simulink model "ieee80211n"  (Simulink 6.0)
settings: Solver=VariableStepDiscrete  StartTime=0.0  StopTime=inf  RelTol=1e-3
PreLoadFcn:
  | load IEEE80211n_init;
values from neighbouring files (symbols this model uses):
  params =     [IEEE80211n_init.mat]    (also in IEEE80211n_settings.m = p)
undefined symbols (not defined in the file or in its folder): magnitude
libraries: commblkintrlv2 x196, dspsigops x143, simulink x136, commdigbbndam2 x98, dspmtrx3 x96, dspsigattribs x69, dspstat3 x38, commutil2 x32, commsequence2 x26, commcnvcod2 x10, dspindex x9, dspmlti3 x8
(part 12 of 12)

== system ieee80211n/MIMODetection/Channel Estimation/ChannelEst6/Channel estimates ==
  trn : Inport  Port=1  LatchInput=off
  in : Inport  Port=2  LatchInput=off
  Enable Averaging : MultiPortSwitch  Inputs=2  zeroidx=on  SaturateOnIntegerOverflow=on
  Enable Averaging1 : MultiPortSwitch  Inputs=2  zeroidx=on  SaturateOnIntegerOverflow=on
  Frame Status Conversion1 : dspsigattribs/Frame Status Conversion  growRefPort=off  outframe=Frame-based
  Mean2 : dspstat3/Mean  DialogController=dspDDGCreate  DialogControllerArgs=DataTag27  run=off  reset_popup=None  roundingMode=Floor  overflowMode=off
  Mean3 : dspstat3/Mean  DialogController=dspDDGCreate  DialogControllerArgs=DataTag28  run=off  reset_popup=None  roundingMode=Floor  overflowMode=off
  Nsts > 1 : Constant  Value=params.NSTS > 1
  One sym only (in) : S-Function  AncestorBlock=dspindex/Multiport Selector  FunctionName=sdspmultiportsel  Parameters=rowsOrCols, numOutports, flatIdxVect, flatLenVect, idxErrMode  mask(Multiport Selector){rowsOrCols=Rows, idxCellArray=1, idxErrMode=Clip Index}
      mask prompts: rowsOrCols "Select:"; idxCellArray "Indices to output:"; idxErrMode "Invalid index:"
      mask help: Output specified rows or columns to one or more output ports. The number of output ports is determined by the number of index vectors, each specified as a separate vector entry in a cell array. Indices are 1-based and need not be unique.
      mask init:
      | [numOutports, flatLenVect, flatIdxVect] = dspblkmultiportsel(idxCellArray);
      mask Help: web(dspbhelp);
      mask StyleString: popup(Rows|Columns),edit,popup(Clip Index|Clip and Warn|Generate Error)
      mask Display: disp(['Select\n' &1]);
  One sym only (trn) : S-Function  AncestorBlock=dspindex/Multiport Selector  FunctionName=sdspmultiportsel  Parameters=rowsOrCols, numOutports, flatIdxVect, flatLenVect, idxErrMode  mask(Multiport Selector){rowsOrCols=Rows, idxCellArray=1, idxErrMode=Clip Index}
      mask prompts: rowsOrCols "Select:"; idxCellArray "Indices to output:"; idxErrMode "Invalid index:"
      mask help: Output specified rows or columns to one or more output ports. The number of output ports is determined by the number of index vectors, each specified as a separate vector entry in a cell array. Indices are 1-based and need not be unique.
      mask init:
      | [numOutports, flatLenVect, flatIdxVect] = dspblkmultiportsel(idxCellArray);
      mask Help: web(dspbhelp);
      mask StyleString: popup(Rows|Columns),edit,popup(Clip Index|Clip and Warn|Generate Error)
      mask Display: disp(['Select\n' &1]);
  Product2 : Product  Inputs=**  SaturateOnIntegerOverflow=on
  Product4 : Product  Inputs=/*  SaturateOnIntegerOverflow=on
  Transpose : dspmtrx3/Transpose  Hermitian=off  overflowFlag=on
  Transpose1 : dspmtrx3/Transpose  Hermitian=off  overflowFlag=on
  Transpose2 : dspmtrx3/Transpose  Hermitian=off  overflowFlag=on
  ch est : Outport
  wires:
  trn/1 -> Transpose/1
  Product4/1 -> Frame Status Conversion1/1
  Frame Status Conversion1/1 -> Transpose1/1
  Transpose1/1 -> ch est/1
  in/1 -> Transpose2/1
  Mean2/1 -> Enable Averaging/3
  Mean3/1 -> Enable Averaging1/3
  Transpose/1 -> Product2/1, Product2/2
  Transpose2/1 -> Mean3/1, One sym only (in)/1
  Product2/1 -> Mean2/1, One sym only (trn)/1
  Enable Averaging/1 -> Product4/1
  Nsts > 1/1 -> Enable Averaging/1, Enable Averaging1/1
  One sym only (in)/1 -> Enable Averaging1/2
  Enable Averaging1/1 -> Product4/2
  One sym only (trn)/1 -> Enable Averaging/2

== system ieee80211n/MIMODetection/Channel Estimation/ChannelEst7/Channel estimates ==
  trn : Inport  Port=1  LatchInput=off
  in : Inport  Port=2  LatchInput=off
  Enable Averaging : MultiPortSwitch  Inputs=2  zeroidx=on  SaturateOnIntegerOverflow=on
  Enable Averaging1 : MultiPortSwitch  Inputs=2  zeroidx=on  SaturateOnIntegerOverflow=on
  Frame Status Conversion1 : dspsigattribs/Frame Status Conversion  growRefPort=off  outframe=Frame-based
  Mean2 : dspstat3/Mean  DialogController=dspDDGCreate  DialogControllerArgs=DataTag29  run=off  reset_popup=None  roundingMode=Floor  overflowMode=off
  Mean3 : dspstat3/Mean  DialogController=dspDDGCreate  DialogControllerArgs=DataTag30  run=off  reset_popup=None  roundingMode=Floor  overflowMode=off
  Nsts > 1 : Constant  Value=params.NSTS > 1
  One sym only (in) : S-Function  AncestorBlock=dspindex/Multiport Selector  FunctionName=sdspmultiportsel  Parameters=rowsOrCols, numOutports, flatIdxVect, flatLenVect, idxErrMode  mask(Multiport Selector){rowsOrCols=Rows, idxCellArray=1, idxErrMode=Clip Index}
      mask prompts: rowsOrCols "Select:"; idxCellArray "Indices to output:"; idxErrMode "Invalid index:"
      mask help: Output specified rows or columns to one or more output ports. The number of output ports is determined by the number of index vectors, each specified as a separate vector entry in a cell array. Indices are 1-based and need not be unique.
      mask init:
      | [numOutports, flatLenVect, flatIdxVect] = dspblkmultiportsel(idxCellArray);
      mask Help: web(dspbhelp);
      mask StyleString: popup(Rows|Columns),edit,popup(Clip Index|Clip and Warn|Generate Error)
      mask Display: disp(['Select\n' &1]);
  One sym only (trn) : S-Function  AncestorBlock=dspindex/Multiport Selector  FunctionName=sdspmultiportsel  Parameters=rowsOrCols, numOutports, flatIdxVect, flatLenVect, idxErrMode  mask(Multiport Selector){rowsOrCols=Rows, idxCellArray=1, idxErrMode=Clip Index}
      mask prompts: rowsOrCols "Select:"; idxCellArray "Indices to output:"; idxErrMode "Invalid index:"
      mask help: Output specified rows or columns to one or more output ports. The number of output ports is determined by the number of index vectors, each specified as a separate vector entry in a cell array. Indices are 1-based and need not be unique.
      mask init:
      | [numOutports, flatLenVect, flatIdxVect] = dspblkmultiportsel(idxCellArray);
      mask Help: web(dspbhelp);
      mask StyleString: popup(Rows|Columns),edit,popup(Clip Index|Clip and Warn|Generate Error)
      mask Display: disp(['Select\n' &1]);
  Product2 : Product  Inputs=**  SaturateOnIntegerOverflow=on
  Product4 : Product  Inputs=/*  SaturateOnIntegerOverflow=on
  Transpose : dspmtrx3/Transpose  Hermitian=off  overflowFlag=on
  Transpose1 : dspmtrx3/Transpose  Hermitian=off  overflowFlag=on
  Transpose2 : dspmtrx3/Transpose  Hermitian=off  overflowFlag=on
  ch est : Outport
  wires:
  trn/1 -> Transpose/1
  Product4/1 -> Frame Status Conversion1/1
  Frame Status Conversion1/1 -> Transpose1/1
  Transpose1/1 -> ch est/1
  in/1 -> Transpose2/1
  Mean2/1 -> Enable Averaging/3
  Mean3/1 -> Enable Averaging1/3
  Transpose/1 -> Product2/1, Product2/2
  Transpose2/1 -> Mean3/1, One sym only (in)/1
  Product2/1 -> Mean2/1, One sym only (trn)/1
  Enable Averaging/1 -> Product4/1
  Nsts > 1/1 -> Enable Averaging/1, Enable Averaging1/1
  One sym only (in)/1 -> Enable Averaging1/2
  Enable Averaging1/1 -> Product4/2
  One sym only (trn)/1 -> Enable Averaging/2

== system ieee80211n/MIMODetection/Channel Estimation/ChannelEst8/Channel estimates ==
  trn : Inport  Port=1  LatchInput=off
  in : Inport  Port=2  LatchInput=off
  Enable Averaging : MultiPortSwitch  Inputs=2  zeroidx=on  SaturateOnIntegerOverflow=on
  Enable Averaging1 : MultiPortSwitch  Inputs=2  zeroidx=on  SaturateOnIntegerOverflow=on
  Frame Status Conversion1 : dspsigattribs/Frame Status Conversion  growRefPort=off  outframe=Frame-based
  Mean2 : dspstat3/Mean  DialogController=dspDDGCreate  DialogControllerArgs=DataTag31  run=off  reset_popup=None  roundingMode=Floor  overflowMode=off
  Mean3 : dspstat3/Mean  DialogController=dspDDGCreate  DialogControllerArgs=DataTag32  run=off  reset_popup=None  roundingMode=Floor  overflowMode=off
  Nsts > 1 : Constant  Value=params.NSTS > 1
  One sym only (in) : S-Function  AncestorBlock=dspindex/Multiport Selector  FunctionName=sdspmultiportsel  Parameters=rowsOrCols, numOutports, flatIdxVect, flatLenVect, idxErrMode  mask(Multiport Selector){rowsOrCols=Rows, idxCellArray=1, idxErrMode=Clip Index}
      mask prompts: rowsOrCols "Select:"; idxCellArray "Indices to output:"; idxErrMode "Invalid index:"
      mask help: Output specified rows or columns to one or more output ports. The number of output ports is determined by the number of index vectors, each specified as a separate vector entry in a cell array. Indices are 1-based and need not be unique.
      mask init:
      | [numOutports, flatLenVect, flatIdxVect] = dspblkmultiportsel(idxCellArray);
      mask Help: web(dspbhelp);
      mask StyleString: popup(Rows|Columns),edit,popup(Clip Index|Clip and Warn|Generate Error)
      mask Display: disp(['Select\n' &1]);
  One sym only (trn) : S-Function  AncestorBlock=dspindex/Multiport Selector  FunctionName=sdspmultiportsel  Parameters=rowsOrCols, numOutports, flatIdxVect, flatLenVect, idxErrMode  mask(Multiport Selector){rowsOrCols=Rows, idxCellArray=1, idxErrMode=Clip Index}
      mask prompts: rowsOrCols "Select:"; idxCellArray "Indices to output:"; idxErrMode "Invalid index:"
      mask help: Output specified rows or columns to one or more output ports. The number of output ports is determined by the number of index vectors, each specified as a separate vector entry in a cell array. Indices are 1-based and need not be unique.
      mask init:
      | [numOutports, flatLenVect, flatIdxVect] = dspblkmultiportsel(idxCellArray);
      mask Help: web(dspbhelp);
      mask StyleString: popup(Rows|Columns),edit,popup(Clip Index|Clip and Warn|Generate Error)
      mask Display: disp(['Select\n' &1]);
  Product2 : Product  Inputs=**  SaturateOnIntegerOverflow=on
  Product4 : Product  Inputs=/*  SaturateOnIntegerOverflow=on
  Transpose : dspmtrx3/Transpose  Hermitian=off  overflowFlag=on
  Transpose1 : dspmtrx3/Transpose  Hermitian=off  overflowFlag=on
  Transpose2 : dspmtrx3/Transpose  Hermitian=off  overflowFlag=on
  ch est : Outport
  wires:
  trn/1 -> Transpose/1
  Product4/1 -> Frame Status Conversion1/1
  Frame Status Conversion1/1 -> Transpose1/1
  Transpose1/1 -> ch est/1
  in/1 -> Transpose2/1
  Mean2/1 -> Enable Averaging/3
  Mean3/1 -> Enable Averaging1/3
  Transpose/1 -> Product2/1, Product2/2
  Transpose2/1 -> Mean3/1, One sym only (in)/1
  Product2/1 -> Mean2/1, One sym only (trn)/1
  Enable Averaging/1 -> Product4/1
  Nsts > 1/1 -> Enable Averaging/1, Enable Averaging1/1
  One sym only (in)/1 -> Enable Averaging1/2
  Enable Averaging1/1 -> Product4/2
  One sym only (trn)/1 -> Enable Averaging/2

== system ieee80211n/MIMODetection/Channel Estimation/ChannelEst9/Channel estimates ==
  trn : Inport  Port=1  LatchInput=off
  in : Inport  Port=2  LatchInput=off
  Enable Averaging : MultiPortSwitch  Inputs=2  zeroidx=on  SaturateOnIntegerOverflow=on
  Enable Averaging1 : MultiPortSwitch  Inputs=2  zeroidx=on  SaturateOnIntegerOverflow=on
  Frame Status Conversion1 : dspsigattribs/Frame Status Conversion  growRefPort=off  outframe=Frame-based
  Mean2 : dspstat3/Mean  DialogController=dspDDGCreate  DialogControllerArgs=DataTag33  run=off  reset_popup=None  roundingMode=Floor  overflowMode=off
  Mean3 : dspstat3/Mean  DialogController=dspDDGCreate  DialogControllerArgs=DataTag34  run=off  reset_popup=None  roundingMode=Floor  overflowMode=off
  Nsts > 1 : Constant  Value=params.NSTS > 1
  One sym only (in) : S-Function  AncestorBlock=dspindex/Multiport Selector  FunctionName=sdspmultiportsel  Parameters=rowsOrCols, numOutports, flatIdxVect, flatLenVect, idxErrMode  mask(Multiport Selector){rowsOrCols=Rows, idxCellArray=1, idxErrMode=Clip Index}
      mask prompts: rowsOrCols "Select:"; idxCellArray "Indices to output:"; idxErrMode "Invalid index:"
      mask help: Output specified rows or columns to one or more output ports. The number of output ports is determined by the number of index vectors, each specified as a separate vector entry in a cell array. Indices are 1-based and need not be unique.
      mask init:
      | [numOutports, flatLenVect, flatIdxVect] = dspblkmultiportsel(idxCellArray);
      mask Help: web(dspbhelp);
      mask StyleString: popup(Rows|Columns),edit,popup(Clip Index|Clip and Warn|Generate Error)
      mask Display: disp(['Select\n' &1]);
  One sym only (trn) : S-Function  AncestorBlock=dspindex/Multiport Selector  FunctionName=sdspmultiportsel  Parameters=rowsOrCols, numOutports, flatIdxVect, flatLenVect, idxErrMode  mask(Multiport Selector){rowsOrCols=Rows, idxCellArray=1, idxErrMode=Clip Index}
      mask prompts: rowsOrCols "Select:"; idxCellArray "Indices to output:"; idxErrMode "Invalid index:"
      mask help: Output specified rows or columns to one or more output ports. The number of output ports is determined by the number of index vectors, each specified as a separate vector entry in a cell array. Indices are 1-based and need not be unique.
      mask init:
      | [numOutports, flatLenVect, flatIdxVect] = dspblkmultiportsel(idxCellArray);
      mask Help: web(dspbhelp);
      mask StyleString: popup(Rows|Columns),edit,popup(Clip Index|Clip and Warn|Generate Error)
      mask Display: disp(['Select\n' &1]);
  Product2 : Product  Inputs=**  SaturateOnIntegerOverflow=on
  Product4 : Product  Inputs=/*  SaturateOnIntegerOverflow=on
  Transpose : dspmtrx3/Transpose  Hermitian=off  overflowFlag=on
  Transpose1 : dspmtrx3/Transpose  Hermitian=off  overflowFlag=on
  Transpose2 : dspmtrx3/Transpose  Hermitian=off  overflowFlag=on
  ch est : Outport
  wires:
  trn/1 -> Transpose/1
  Product4/1 -> Frame Status Conversion1/1
  Frame Status Conversion1/1 -> Transpose1/1
  Transpose1/1 -> ch est/1
  in/1 -> Transpose2/1
  Mean2/1 -> Enable Averaging/3
  Mean3/1 -> Enable Averaging1/3
  Transpose/1 -> Product2/1, Product2/2
  Transpose2/1 -> Mean3/1, One sym only (in)/1
  Product2/1 -> Mean2/1, One sym only (trn)/1
  Enable Averaging/1 -> Product4/1
  Nsts > 1/1 -> Enable Averaging/1, Enable Averaging1/1
  One sym only (in)/1 -> Enable Averaging1/2
  Enable Averaging1/1 -> Product4/2
  One sym only (trn)/1 -> Enable Averaging/2

== system ieee80211n/ModulatorBank/Group into OFDM symbols/Group into OFDM symbols/DC value ==
  Constant : Constant  Value=complex(zeros(1,params.OFDMSymPerFrame))  VectorParams1D=off
  Frame Status Conversion1 : dspsigattribs/Frame Status Conversion  growRefPort=off  outframe=Frame-based
  out : Outport
  wires:
  Frame Status Conversion1/1 -> out/1
  Constant/1 -> Frame Status Conversion1/1

== system ieee80211n/ModulatorBank/Group into OFDM symbols/Group into OFDM symbols/Pilot1 ==
  Constant : Constant  Value=params.dmPilot1_seq_ss1  VectorParams1D=off
  Frame Status Conversion1 : dspsigattribs/Frame Status Conversion  growRefPort=off  outframe=Frame-based
  out : Outport
  wires:
  Frame Status Conversion1/1 -> out/1
  Constant/1 -> Frame Status Conversion1/1

== system ieee80211n/ModulatorBank/Group into OFDM symbols/Group into OFDM symbols/Pilot2 ==
  Constant : Constant  Value=params.dmPilot2_seq_ss1  VectorParams1D=off
  Frame Status Conversion1 : dspsigattribs/Frame Status Conversion  growRefPort=off  outframe=Frame-based
  out : Outport
  wires:
  Frame Status Conversion1/1 -> out/1
  Constant/1 -> Frame Status Conversion1/1

== system ieee80211n/ModulatorBank/Group into OFDM symbols/Group into OFDM symbols/Pilot3 ==
  Constant : Constant  Value=params.dmPilot3_seq_ss1  VectorParams1D=off
  Frame Status Conversion1 : dspsigattribs/Frame Status Conversion  growRefPort=off  outframe=Frame-based
  out : Outport
  wires:
  Frame Status Conversion1/1 -> out/1
  Constant/1 -> Frame Status Conversion1/1

== system ieee80211n/ModulatorBank/Group into OFDM symbols/Group into OFDM symbols/Pilot4 ==
  Constant : Constant  Value=params.dmPilot4_seq_ss1  VectorParams1D=off
  Frame Status Conversion1 : dspsigattribs/Frame Status Conversion  growRefPort=off  outframe=Frame-based
  out : Outport
  wires:
  Frame Status Conversion1/1 -> out/1
  Constant/1 -> Frame Status Conversion1/1

== system ieee80211n/ModulatorBank/Group into OFDM symbols1/Group into OFDM symbols/DC value ==
  Constant : Constant  Value=complex(zeros(1,params.OFDMSymPerFrame))  VectorParams1D=off
  Frame Status Conversion1 : dspsigattribs/Frame Status Conversion  growRefPort=off  outframe=Frame-based
  out : Outport
  wires:
  Frame Status Conversion1/1 -> out/1
  Constant/1 -> Frame Status Conversion1/1

== system ieee80211n/ModulatorBank/Group into OFDM symbols1/Group into OFDM symbols/Pilot1 ==
  Constant : Constant  Value=params.dmPilot1_seq_ss2  VectorParams1D=off
  Frame Status Conversion1 : dspsigattribs/Frame Status Conversion  growRefPort=off  outframe=Frame-based
  out : Outport
  wires:
  Frame Status Conversion1/1 -> out/1
  Constant/1 -> Frame Status Conversion1/1

== system ieee80211n/ModulatorBank/Group into OFDM symbols1/Group into OFDM symbols/Pilot2 ==
  Constant : Constant  Value=params.dmPilot2_seq_ss2  VectorParams1D=off
  Frame Status Conversion1 : dspsigattribs/Frame Status Conversion  growRefPort=off  outframe=Frame-based
  out : Outport
  wires:
  Frame Status Conversion1/1 -> out/1
  Constant/1 -> Frame Status Conversion1/1

== system ieee80211n/ModulatorBank/Group into OFDM symbols1/Group into OFDM symbols/Pilot3 ==
  Constant : Constant  Value=params.dmPilot3_seq_ss2  VectorParams1D=off
  Frame Status Conversion1 : dspsigattribs/Frame Status Conversion  growRefPort=off  outframe=Frame-based
  out : Outport
  wires:
  Frame Status Conversion1/1 -> out/1
  Constant/1 -> Frame Status Conversion1/1

== system ieee80211n/ModulatorBank/Group into OFDM symbols1/Group into OFDM symbols/Pilot4 ==
  Constant : Constant  Value=params.dmPilot4_seq_ss2  VectorParams1D=off
  Frame Status Conversion1 : dspsigattribs/Frame Status Conversion  growRefPort=off  outframe=Frame-based
  out : Outport
  wires:
  Frame Status Conversion1/1 -> out/1
  Constant/1 -> Frame Status Conversion1/1

== system ieee80211n/ModulatorBank/Group into OFDM symbols2/Group into OFDM symbols/DC value ==
  Constant : Constant  Value=complex(zeros(1,params.OFDMSymPerFrame))  VectorParams1D=off
  Frame Status Conversion1 : dspsigattribs/Frame Status Conversion  growRefPort=off  outframe=Frame-based
  out : Outport
  wires:
  Frame Status Conversion1/1 -> out/1
  Constant/1 -> Frame Status Conversion1/1

== system ieee80211n/ModulatorBank/Group into OFDM symbols2/Group into OFDM symbols/Pilot1 ==
  Constant : Constant  Value=params.dmPilot1_seq_ss3  VectorParams1D=off
  Frame Status Conversion1 : dspsigattribs/Frame Status Conversion  growRefPort=off  outframe=Frame-based
  out : Outport
  wires:
  Frame Status Conversion1/1 -> out/1
  Constant/1 -> Frame Status Conversion1/1

== system ieee80211n/ModulatorBank/Group into OFDM symbols2/Group into OFDM symbols/Pilot2 ==
  Constant : Constant  Value=params.dmPilot2_seq_ss3  VectorParams1D=off
  Frame Status Conversion1 : dspsigattribs/Frame Status Conversion  growRefPort=off  outframe=Frame-based
  out : Outport
  wires:
  Frame Status Conversion1/1 -> out/1
  Constant/1 -> Frame Status Conversion1/1

== system ieee80211n/ModulatorBank/Group into OFDM symbols2/Group into OFDM symbols/Pilot3 ==
  Constant : Constant  Value=params.dmPilot3_seq_ss3  VectorParams1D=off
  Frame Status Conversion1 : dspsigattribs/Frame Status Conversion  growRefPort=off  outframe=Frame-based
  out : Outport
  wires:
  Frame Status Conversion1/1 -> out/1
  Constant/1 -> Frame Status Conversion1/1

== system ieee80211n/ModulatorBank/Group into OFDM symbols2/Group into OFDM symbols/Pilot4 ==
  Constant : Constant  Value=params.dmPilot4_seq_ss3  VectorParams1D=off
  Frame Status Conversion1 : dspsigattribs/Frame Status Conversion  growRefPort=off  outframe=Frame-based
  out : Outport
  wires:
  Frame Status Conversion1/1 -> out/1
  Constant/1 -> Frame Status Conversion1/1

== system ieee80211n/ModulatorBank/Group into OFDM symbols3/Group into OFDM symbols/DC value ==
  Constant : Constant  Value=complex(zeros(1,params.OFDMSymPerFrame))  VectorParams1D=off
  Frame Status Conversion1 : dspsigattribs/Frame Status Conversion  growRefPort=off  outframe=Frame-based
  out : Outport
  wires:
  Frame Status Conversion1/1 -> out/1
  Constant/1 -> Frame Status Conversion1/1

== system ieee80211n/ModulatorBank/Group into OFDM symbols3/Group into OFDM symbols/Pilot1 ==
  Constant : Constant  Value=params.dmPilot1_seq_ss4  VectorParams1D=off
  Frame Status Conversion1 : dspsigattribs/Frame Status Conversion  growRefPort=off  outframe=Frame-based
  out : Outport
  wires:
  Frame Status Conversion1/1 -> out/1
  Constant/1 -> Frame Status Conversion1/1

== system ieee80211n/ModulatorBank/Group into OFDM symbols3/Group into OFDM symbols/Pilot2 ==
  Constant : Constant  Value=params.dmPilot2_seq_ss4  VectorParams1D=off
  Frame Status Conversion1 : dspsigattribs/Frame Status Conversion  growRefPort=off  outframe=Frame-based
  out : Outport
  wires:
  Frame Status Conversion1/1 -> out/1
  Constant/1 -> Frame Status Conversion1/1

== system ieee80211n/ModulatorBank/Group into OFDM symbols3/Group into OFDM symbols/Pilot3 ==
  Constant : Constant  Value=params.dmPilot3_seq_ss4  VectorParams1D=off
  Frame Status Conversion1 : dspsigattribs/Frame Status Conversion  growRefPort=off  outframe=Frame-based
  out : Outport
  wires:
  Frame Status Conversion1/1 -> out/1
  Constant/1 -> Frame Status Conversion1/1

== system ieee80211n/ModulatorBank/Group into OFDM symbols3/Group into OFDM symbols/Pilot4 ==
  Constant : Constant  Value=params.dmPilot4_seq_ss4  VectorParams1D=off
  Frame Status Conversion1 : dspsigattribs/Frame Status Conversion  growRefPort=off  outframe=Frame-based
  out : Outport
  wires:
  Frame Status Conversion1/1 -> out/1
  Constant/1 -> Frame Status Conversion1/1

== system ieee80211n/training sequence4/Modulator/Group into OFDM symbols/DC value ==
  Constant : Constant  Value=complex(zeros(1,params.OFDM_LSIG_SymPerFrame))  VectorParams1D=off
  Frame Status Conversion4 : dspsigattribs/Frame Status Conversion  growRefPort=off  outframe=Frame-based
  out : Outport
  wires:
  Frame Status Conversion4/1 -> out/1
  Constant/1 -> Frame Status Conversion4/1

== system ieee80211n/training sequence4/Modulator/Group into OFDM symbols/DC value1 ==
  Constant : Constant  Value=complex(zeros(2,params.OFDM_LSIG_SymPerFrame))  VectorParams1D=off
  Frame Status Conversion4 : dspsigattribs/Frame Status Conversion  growRefPort=off  outframe=Frame-based
  out : Outport
  wires:
  Frame Status Conversion4/1 -> out/1
  Constant/1 -> Frame Status Conversion4/1

== system ieee80211n/training sequence4/Modulator/Group into OFDM symbols/DC value2 ==
  Constant : Constant  Value=complex(zeros(2,params.OFDM_LSIG_SymPerFrame))  VectorParams1D=off
  Frame Status Conversion4 : dspsigattribs/Frame Status Conversion  growRefPort=off  outframe=Frame-based
  out : Outport
  wires:
  Frame Status Conversion4/1 -> out/1
  Constant/1 -> Frame Status Conversion4/1

== system ieee80211n/training sequence4/Modulator1/Group into OFDM symbols/DC value ==
  Constant : Constant  Value=complex(zeros(1,params.OFDM_HTSIG_SymPerFrame))  VectorParams1D=off
  Frame Status Conversion4 : dspsigattribs/Frame Status Conversion  growRefPort=off  outframe=Frame-based
  out : Outport
  wires:
  Frame Status Conversion4/1 -> out/1
  Constant/1 -> Frame Status Conversion4/1

== system ieee80211n/training sequence4/Modulator1/Group into OFDM symbols/DC value1 ==
  Constant : Constant  Value=complex(zeros(2,params.OFDM_HTSIG_SymPerFrame))  VectorParams1D=off
  Frame Status Conversion4 : dspsigattribs/Frame Status Conversion  growRefPort=off  outframe=Frame-based
  out : Outport
  wires:
  Frame Status Conversion4/1 -> out/1
  Constant/1 -> Frame Status Conversion4/1

== system ieee80211n/training sequence4/Modulator1/Group into OFDM symbols/DC value2 ==
  Constant : Constant  Value=complex(zeros(2,params.OFDM_HTSIG_SymPerFrame))  VectorParams1D=off
  Frame Status Conversion4 : dspsigattribs/Frame Status Conversion  growRefPort=off  outframe=Frame-based
  out : Outport
  wires:
  Frame Status Conversion4/1 -> out/1
  Constant/1 -> Frame Status Conversion4/1
